simulink model "TST_CrCtl_Governor"  (R2016b)
settings: Solver=FixedStepDiscrete  StartTime=0.0  StopTime=simTime  FixedStep=sampleTime  RelTol=1e-3
values from neighbouring files (symbols this model uses):
  testCase = 1    [initTST_CrCtl_Governor_001.m]    (also in initTST_CrCtl_Governor_002.m = 2; initTST_CrCtl_Governor_003.m = 3; initTST_CrCtl_Governor_004.m = 4; initTST_CrCtl_Governor_005.m = 5)
libraries: simulink x144, UnitTest_Lib x110
(part 7 of 7)

== system TST_CrCtl_Governor/compareSignals/Requirement_002/specifyOutputs ==
  sig_Req_Bus : Inport
  sig_Result_Bus : Inport  Port=2
  AndN : Logic  Inputs=12
  BS_Req : BusSelector  OutputSignals=testSig_CrCtl_rTraV2NBeg,testSig_CrCtl_stOpFunc,testSig_CrCtl_stPtd,testSig_CrCtl_stReq,testSig_CrCtl_stSuspRamp,testSig_CrCtl_stvHysEngBrkReq,testSig_CrCtl_trqLead,testSig_CrCtl_trqLimAct,testSig_CrCtl_trqMin,testSig_CrCtl_trqReq,testSig_CrCtl_trqReqOld,testSig_CrCtl_vMax
  BS_Result : BusSelector  OutputSignals=CrCtl_rTraV2NBeg,CrCtl_stOpFunc,CrCtl_stPtd,CrCtl_stReq,CrCtl_stSuspRamp,CrCtl_stvHysEngBrkReq,CrCtl_trqLead,CrCtl_trqLimAct,CrCtl_trqMin,CrCtl_trqReq,CrCtl_trqReqOld,CrCtl_vMax
  Bitwise_And{1..12} (12 alike) : simulink/Logic and Bit Operations/Bitwise Operator  logicop=AND  UseBitMask=off  BitMask=bin2dec('11011001')  BitMaskRealWorld=Stored Integer
  Relational Operator1 : RelationalOperator  Operator===  OutDataTypeStr=boolean  RndMeth=Simplest
  Relational Operator2 : RelationalOperator  Operator===  OutDataTypeStr=boolean  RndMeth=Simplest
  Scope : Scope  NumInputPorts=12
  Scope{1..12} (12 alike) : Scope  NumInputPorts=2
  cmp_{1,3..4,6..12} (10 alike) : UnitTest_Lib/RoughlyEqual  slope=0.1
  result_tws : ToWorkspace  VariableName=spec_result_002
  tws_1 : ToWorkspace  VariableName=spec_req_002_001
  tws_10 : ToWorkspace  VariableName=spec_req_002_010
  tws_11 : ToWorkspace  VariableName=spec_req_002_011
  tws_12 : ToWorkspace  VariableName=spec_req_002_012
  tws_2 : ToWorkspace  VariableName=spec_req_002_002
  tws_3 : ToWorkspace  VariableName=spec_req_002_003
  tws_4 : ToWorkspace  VariableName=spec_req_002_004
  tws_5 : ToWorkspace  VariableName=spec_req_002_005
  tws_6 : ToWorkspace  VariableName=spec_req_002_006
  tws_7 : ToWorkspace  VariableName=spec_req_002_007
  tws_8 : ToWorkspace  VariableName=spec_req_002_008
  tws_9 : ToWorkspace  VariableName=spec_req_002_009
  result : Outport
  wires:
  sig_Req_Bus/1 -> BS_Req/1
  sig_Result_Bus/1 -> BS_Result/1
  AndN/1 -> result/1, result_tws/1
  BS_Req/1 -> cmp_1/1, Scope1/1  "<testSig_CrCtl_rTraV2NBeg>"
  BS_Result/1 -> cmp_1/2, Scope1/2  "<CrCtl_rTraV2NBeg>"
  cmp_1/1 -> Bitwise_And1/1
  Bitwise_And1/1 -> AndN/1, Scope/1, tws_1/1
  BS_Req/2 -> Relational Operator1/1, Scope2/1  "<testSig_CrCtl_stOpFunc>"
  BS_Result/2 -> Scope2/2, Relational Operator1/2  "<CrCtl_stOpFunc>"
  Relational Operator1/1 -> Bitwise_And2/1
  Bitwise_And2/1 -> AndN/2, Scope/2, tws_2/1
  BS_Req/3 -> cmp_3/1, Scope3/1  "<testSig_CrCtl_stPtd>"
  BS_Result/3 -> cmp_3/2, Scope3/2  "<CrCtl_stPtd>"
  cmp_3/1 -> Bitwise_And3/1
  Bitwise_And3/1 -> AndN/3, Scope/3, tws_3/1
  BS_Req/4 -> cmp_4/1, Scope4/1  "<testSig_CrCtl_stReq>"
  BS_Result/4 -> cmp_4/2, Scope4/2  "<CrCtl_stReq>"
  cmp_4/1 -> Bitwise_And4/1
  Bitwise_And4/1 -> AndN/4, Scope/4, tws_4/1
  BS_Req/5 -> Relational Operator2/1, Scope5/1  "<testSig_CrCtl_stSuspRamp>"
  BS_Result/5 -> Scope5/2, Relational Operator2/2  "<CrCtl_stSuspRamp>"
  Relational Operator2/1 -> Bitwise_And5/1
  Bitwise_And5/1 -> AndN/5, Scope/5, tws_5/1
  BS_Req/6 -> cmp_6/1, Scope6/1  "<testSig_CrCtl_stvHysEngBrkReq>"
  BS_Result/6 -> cmp_6/2, Scope6/2  "<CrCtl_stvHysEngBrkReq>"
  cmp_6/1 -> Bitwise_And6/1
  Bitwise_And6/1 -> AndN/6, Scope/6, tws_6/1
  BS_Req/7 -> cmp_7/1, Scope7/1  "<testSig_CrCtl_trqLead>"
  BS_Result/7 -> cmp_7/2, Scope7/2  "<CrCtl_trqLead>"
  cmp_7/1 -> Bitwise_And7/1
  Bitwise_And7/1 -> AndN/7, Scope/7, tws_7/1
  BS_Req/8 -> cmp_8/1, Scope8/1  "<testSig_CrCtl_trqLimAct>"
  BS_Result/8 -> cmp_8/2, Scope8/2  "<CrCtl_trqLimAct>"
  cmp_8/1 -> Bitwise_And8/1
  Bitwise_And8/1 -> AndN/8, Scope/8, tws_8/1
  BS_Req/9 -> cmp_9/1, Scope9/1  "<testSig_CrCtl_trqMin>"
  BS_Result/9 -> cmp_9/2, Scope9/2  "<CrCtl_trqMin>"
  cmp_9/1 -> Bitwise_And9/1
  Bitwise_And9/1 -> AndN/9, Scope/9, tws_9/1
  BS_Req/10 -> cmp_10/1, Scope10/1  "<testSig_CrCtl_trqReq>"
  BS_Result/10 -> cmp_10/2, Scope10/2  "<CrCtl_trqReq>"
  cmp_10/1 -> Bitwise_And10/1
  Bitwise_And10/1 -> AndN/10, Scope/10, tws_10/1
  BS_Req/11 -> cmp_11/1, Scope11/1  "<testSig_CrCtl_trqReqOld>"
  BS_Result/11 -> cmp_11/2, Scope11/2  "<CrCtl_trqReqOld>"
  cmp_11/1 -> Bitwise_And11/1
  Bitwise_And11/1 -> AndN/11, Scope/11, tws_11/1
  BS_Req/12 -> cmp_12/1, Scope12/1  "<testSig_CrCtl_vMax>"
  BS_Result/12 -> cmp_12/2, Scope12/2  "<CrCtl_vMax>"
  cmp_12/1 -> Bitwise_And12/1
  Bitwise_And12/1 -> AndN/12, Scope/12, tws_12/1

== system TST_CrCtl_Governor/compareSignals/Requirement_003/specifyOutputs ==
  sig_Req_Bus : Inport
  sig_Result_Bus : Inport  Port=2
  AndN : Logic  Inputs=12
  BS_Req : BusSelector  OutputSignals=testSig_CrCtl_rTraV2NBeg,testSig_CrCtl_stOpFunc,testSig_CrCtl_stPtd,testSig_CrCtl_stReq,testSig_CrCtl_stSuspRamp,testSig_CrCtl_stvHysEngBrkReq,testSig_CrCtl_trqLead,testSig_CrCtl_trqLimAct,testSig_CrCtl_trqMin,testSig_CrCtl_trqReq,testSig_CrCtl_trqReqOld,testSig_CrCtl_vMax
  BS_Result : BusSelector  OutputSignals=CrCtl_rTraV2NBeg,CrCtl_stOpFunc,CrCtl_stPtd,CrCtl_stReq,CrCtl_stSuspRamp,CrCtl_stvHysEngBrkReq,CrCtl_trqLead,CrCtl_trqLimAct,CrCtl_trqMin,CrCtl_trqReq,CrCtl_trqReqOld,CrCtl_vMax
  Bitwise_And{1..12} (12 alike) : simulink/Logic and Bit Operations/Bitwise Operator  logicop=AND  UseBitMask=off  BitMask=bin2dec('11011001')  BitMaskRealWorld=Stored Integer
  Relational Operator1 : RelationalOperator  Operator===  OutDataTypeStr=boolean  RndMeth=Simplest
  Relational Operator2 : RelationalOperator  Operator===  OutDataTypeStr=boolean  RndMeth=Simplest
  Scope : Scope  NumInputPorts=12
  Scope{1..12} (12 alike) : Scope  NumInputPorts=2
  cmp_{1,3..4,6..12} (10 alike) : UnitTest_Lib/RoughlyEqual  slope=0.1
  result_tws : ToWorkspace  VariableName=spec_result_003
  tws_1 : ToWorkspace  VariableName=spec_req_003_001
  tws_10 : ToWorkspace  VariableName=spec_req_003_010
  tws_11 : ToWorkspace  VariableName=spec_req_003_011
  tws_12 : ToWorkspace  VariableName=spec_req_003_012
  tws_2 : ToWorkspace  VariableName=spec_req_003_002
  tws_3 : ToWorkspace  VariableName=spec_req_003_003
  tws_4 : ToWorkspace  VariableName=spec_req_003_004
  tws_5 : ToWorkspace  VariableName=spec_req_003_005
  tws_6 : ToWorkspace  VariableName=spec_req_003_006
  tws_7 : ToWorkspace  VariableName=spec_req_003_007
  tws_8 : ToWorkspace  VariableName=spec_req_003_008
  tws_9 : ToWorkspace  VariableName=spec_req_003_009
  result : Outport
  wires:
  sig_Req_Bus/1 -> BS_Req/1
  sig_Result_Bus/1 -> BS_Result/1
  AndN/1 -> result/1, result_tws/1
  BS_Req/1 -> cmp_1/1, Scope1/1  "<testSig_CrCtl_rTraV2NBeg>"
  BS_Result/1 -> cmp_1/2, Scope1/2  "<CrCtl_rTraV2NBeg>"
  cmp_1/1 -> Bitwise_And1/1
  Bitwise_And1/1 -> AndN/1, Scope/1, tws_1/1
  BS_Req/2 -> Relational Operator1/1, Scope2/1  "<testSig_CrCtl_stOpFunc>"
  BS_Result/2 -> Scope2/2, Relational Operator1/2  "<CrCtl_stOpFunc>"
  Relational Operator1/1 -> Bitwise_And2/1
  Bitwise_And2/1 -> AndN/2, Scope/2, tws_2/1
  BS_Req/3 -> cmp_3/1, Scope3/1  "<testSig_CrCtl_stPtd>"
  BS_Result/3 -> cmp_3/2, Scope3/2  "<CrCtl_stPtd>"
  cmp_3/1 -> Bitwise_And3/1
  Bitwise_And3/1 -> AndN/3, Scope/3, tws_3/1
  BS_Req/4 -> cmp_4/1, Scope4/1  "<testSig_CrCtl_stReq>"
  BS_Result/4 -> cmp_4/2, Scope4/2  "<CrCtl_stReq>"
  cmp_4/1 -> Bitwise_And4/1
  Bitwise_And4/1 -> AndN/4, Scope/4, tws_4/1
  BS_Req/5 -> Relational Operator2/1, Scope5/1  "<testSig_CrCtl_stSuspRamp>"
  BS_Result/5 -> Scope5/2, Relational Operator2/2  "<CrCtl_stSuspRamp>"
  Relational Operator2/1 -> Bitwise_And5/1
  Bitwise_And5/1 -> AndN/5, Scope/5, tws_5/1
  BS_Req/6 -> cmp_6/1, Scope6/1  "<testSig_CrCtl_stvHysEngBrkReq>"
  BS_Result/6 -> cmp_6/2, Scope6/2  "<CrCtl_stvHysEngBrkReq>"
  cmp_6/1 -> Bitwise_And6/1
  Bitwise_And6/1 -> AndN/6, Scope/6, tws_6/1
  BS_Req/7 -> cmp_7/1, Scope7/1  "<testSig_CrCtl_trqLead>"
  BS_Result/7 -> cmp_7/2, Scope7/2  "<CrCtl_trqLead>"
  cmp_7/1 -> Bitwise_And7/1
  Bitwise_And7/1 -> AndN/7, Scope/7, tws_7/1
  BS_Req/8 -> cmp_8/1, Scope8/1  "<testSig_CrCtl_trqLimAct>"
  BS_Result/8 -> cmp_8/2, Scope8/2  "<CrCtl_trqLimAct>"
  cmp_8/1 -> Bitwise_And8/1
  Bitwise_And8/1 -> AndN/8, Scope/8, tws_8/1
  BS_Req/9 -> cmp_9/1, Scope9/1  "<testSig_CrCtl_trqMin>"
  BS_Result/9 -> cmp_9/2, Scope9/2  "<CrCtl_trqMin>"
  cmp_9/1 -> Bitwise_And9/1
  Bitwise_And9/1 -> AndN/9, Scope/9, tws_9/1
  BS_Req/10 -> cmp_10/1, Scope10/1  "<testSig_CrCtl_trqReq>"
  BS_Result/10 -> cmp_10/2, Scope10/2  "<CrCtl_trqReq>"
  cmp_10/1 -> Bitwise_And10/1
  Bitwise_And10/1 -> AndN/10, Scope/10, tws_10/1
  BS_Req/11 -> cmp_11/1, Scope11/1  "<testSig_CrCtl_trqReqOld>"
  BS_Result/11 -> cmp_11/2, Scope11/2  "<CrCtl_trqReqOld>"
  cmp_11/1 -> Bitwise_And11/1
  Bitwise_And11/1 -> AndN/11, Scope/11, tws_11/1
  BS_Req/12 -> cmp_12/1, Scope12/1  "<testSig_CrCtl_vMax>"
  BS_Result/12 -> cmp_12/2, Scope12/2  "<CrCtl_vMax>"
  cmp_12/1 -> Bitwise_And12/1
  Bitwise_And12/1 -> AndN/12, Scope/12, tws_12/1

== system TST_CrCtl_Governor/compareSignals/Requirement_004/specifyOutputs ==
  sig_Req_Bus : Inport
  sig_Result_Bus : Inport  Port=2
  AndN : Logic  Inputs=12
  BS_Req : BusSelector  OutputSignals=testSig_CrCtl_rTraV2NBeg,testSig_CrCtl_stOpFunc,testSig_CrCtl_stPtd,testSig_CrCtl_stReq,testSig_CrCtl_stSuspRamp,testSig_CrCtl_stvHysEngBrkReq,testSig_CrCtl_trqLead,testSig_CrCtl_trqLimAct,testSig_CrCtl_trqMin,testSig_CrCtl_trqReq,testSig_CrCtl_trqReqOld,testSig_CrCtl_vMax
  BS_Result : BusSelector  OutputSignals=CrCtl_rTraV2NBeg,CrCtl_stOpFunc,CrCtl_stPtd,CrCtl_stReq,CrCtl_stSuspRamp,CrCtl_stvHysEngBrkReq,CrCtl_trqLead,CrCtl_trqLimAct,CrCtl_trqMin,CrCtl_trqReq,CrCtl_trqReqOld,CrCtl_vMax
  Bitwise_And{1..12} (12 alike) : simulink/Logic and Bit Operations/Bitwise Operator  logicop=AND  UseBitMask=off  BitMask=bin2dec('11011001')  BitMaskRealWorld=Stored Integer
  Relational Operator1 : RelationalOperator  Operator===  OutDataTypeStr=boolean  RndMeth=Simplest
  Relational Operator2 : RelationalOperator  Operator===  OutDataTypeStr=boolean  RndMeth=Simplest
  Scope : Scope  NumInputPorts=12
  Scope{1..12} (12 alike) : Scope  NumInputPorts=2
  cmp_{1,3..4,6..12} (10 alike) : UnitTest_Lib/RoughlyEqual  slope=0.1
  result_tws : ToWorkspace  VariableName=spec_result_004
  tws_1 : ToWorkspace  VariableName=spec_req_004_001
  tws_10 : ToWorkspace  VariableName=spec_req_004_010
  tws_11 : ToWorkspace  VariableName=spec_req_004_011
  tws_12 : ToWorkspace  VariableName=spec_req_004_012
  tws_2 : ToWorkspace  VariableName=spec_req_004_002
  tws_3 : ToWorkspace  VariableName=spec_req_004_003
  tws_4 : ToWorkspace  VariableName=spec_req_004_004
  tws_5 : ToWorkspace  VariableName=spec_req_004_005
  tws_6 : ToWorkspace  VariableName=spec_req_004_006
  tws_7 : ToWorkspace  VariableName=spec_req_004_007
  tws_8 : ToWorkspace  VariableName=spec_req_004_008
  tws_9 : ToWorkspace  VariableName=spec_req_004_009
  result : Outport
  wires:
  sig_Req_Bus/1 -> BS_Req/1
  sig_Result_Bus/1 -> BS_Result/1
  AndN/1 -> result/1, result_tws/1
  BS_Req/1 -> cmp_1/1, Scope1/1  "<testSig_CrCtl_rTraV2NBeg>"
  BS_Result/1 -> cmp_1/2, Scope1/2  "<CrCtl_rTraV2NBeg>"
  cmp_1/1 -> Bitwise_And1/1
  Bitwise_And1/1 -> AndN/1, Scope/1, tws_1/1
  BS_Req/2 -> Relational Operator1/1, Scope2/1  "<testSig_CrCtl_stOpFunc>"
  BS_Result/2 -> Relational Operator1/2, Scope2/2  "<CrCtl_stOpFunc>"
  Relational Operator1/1 -> Bitwise_And2/1
  Bitwise_And2/1 -> AndN/2, Scope/2, tws_2/1
  BS_Req/3 -> cmp_3/1, Scope3/1  "<testSig_CrCtl_stPtd>"
  BS_Result/3 -> cmp_3/2, Scope3/2  "<CrCtl_stPtd>"
  cmp_3/1 -> Bitwise_And3/1
  Bitwise_And3/1 -> AndN/3, Scope/3, tws_3/1
  BS_Req/4 -> cmp_4/1, Scope4/1  "<testSig_CrCtl_stReq>"
  BS_Result/4 -> cmp_4/2, Scope4/2  "<CrCtl_stReq>"
  cmp_4/1 -> Bitwise_And4/1
  Bitwise_And4/1 -> AndN/4, Scope/4, tws_4/1
  BS_Req/5 -> Relational Operator2/1, Scope5/1  "<testSig_CrCtl_stSuspRamp>"
  BS_Result/5 -> Scope5/2, Relational Operator2/2  "<CrCtl_stSuspRamp>"
  Relational Operator2/1 -> Bitwise_And5/1
  Bitwise_And5/1 -> AndN/5, Scope/5, tws_5/1
  BS_Req/6 -> cmp_6/1, Scope6/1  "<testSig_CrCtl_stvHysEngBrkReq>"
  BS_Result/6 -> cmp_6/2, Scope6/2  "<CrCtl_stvHysEngBrkReq>"
  cmp_6/1 -> Bitwise_And6/1
  Bitwise_And6/1 -> AndN/6, Scope/6, tws_6/1
  BS_Req/7 -> cmp_7/1, Scope7/1  "<testSig_CrCtl_trqLead>"
  BS_Result/7 -> cmp_7/2, Scope7/2  "<CrCtl_trqLead>"
  cmp_7/1 -> Bitwise_And7/1
  Bitwise_And7/1 -> AndN/7, Scope/7, tws_7/1
  BS_Req/8 -> cmp_8/1, Scope8/1  "<testSig_CrCtl_trqLimAct>"
  BS_Result/8 -> cmp_8/2, Scope8/2  "<CrCtl_trqLimAct>"
  cmp_8/1 -> Bitwise_And8/1
  Bitwise_And8/1 -> AndN/8, Scope/8, tws_8/1
  BS_Req/9 -> cmp_9/1, Scope9/1  "<testSig_CrCtl_trqMin>"
  BS_Result/9 -> cmp_9/2, Scope9/2  "<CrCtl_trqMin>"
  cmp_9/1 -> Bitwise_And9/1
  Bitwise_And9/1 -> AndN/9, Scope/9, tws_9/1
  BS_Req/10 -> cmp_10/1, Scope10/1  "<testSig_CrCtl_trqReq>"
  BS_Result/10 -> cmp_10/2, Scope10/2  "<CrCtl_trqReq>"
  cmp_10/1 -> Bitwise_And10/1
  Bitwise_And10/1 -> AndN/10, Scope/10, tws_10/1
  BS_Req/11 -> cmp_11/1, Scope11/1  "<testSig_CrCtl_trqReqOld>"
  BS_Result/11 -> cmp_11/2, Scope11/2  "<CrCtl_trqReqOld>"
  cmp_11/1 -> Bitwise_And11/1
  Bitwise_And11/1 -> AndN/11, Scope/11, tws_11/1
  BS_Req/12 -> cmp_12/1, Scope12/1  "<testSig_CrCtl_vMax>"
  BS_Result/12 -> cmp_12/2, Scope12/2  "<CrCtl_vMax>"
  cmp_12/1 -> Bitwise_And12/1
  Bitwise_And12/1 -> AndN/12, Scope/12, tws_12/1

== system TST_CrCtl_Governor/compareSignals/Requirement_005/specifyOutputs ==
  sig_Req_Bus : Inport
  sig_Result_Bus : Inport  Port=2
  AndN : Logic  Inputs=12
  BS_Req : BusSelector  OutputSignals=testSig_CrCtl_rTraV2NBeg,testSig_CrCtl_stOpFunc,testSig_CrCtl_stPtd,testSig_CrCtl_stReq,testSig_CrCtl_stSuspRamp,testSig_CrCtl_stvHysEngBrkReq,testSig_CrCtl_trqLead,testSig_CrCtl_trqLimAct,testSig_CrCtl_trqMin,testSig_CrCtl_trqReq,testSig_CrCtl_trqReqOld,testSig_CrCtl_vMax
  BS_Result : BusSelector  OutputSignals=CrCtl_rTraV2NBeg,CrCtl_stOpFunc,CrCtl_stPtd,CrCtl_stReq,CrCtl_stSuspRamp,CrCtl_stvHysEngBrkReq,CrCtl_trqLead,CrCtl_trqLimAct,CrCtl_trqMin,CrCtl_trqReq,CrCtl_trqReqOld,CrCtl_vMax
  Bitwise_And{1..12} (12 alike) : simulink/Logic and Bit Operations/Bitwise Operator  logicop=AND  UseBitMask=off  BitMask=bin2dec('11011001')  BitMaskRealWorld=Stored Integer
  Relational Operator1 : RelationalOperator  Operator===  OutDataTypeStr=boolean  RndMeth=Simplest
  Relational Operator2 : RelationalOperator  Operator===  OutDataTypeStr=boolean  RndMeth=Simplest
  Scope : Scope  NumInputPorts=12
  Scope{1..12} (12 alike) : Scope  NumInputPorts=2
  cmp_{1,3..4,6..9,12} (8 alike) : UnitTest_Lib/RoughlyEqual  slope=0.1
  cmp_10 : UnitTest_Lib/RoughlyEqual  slope=0.5
  cmp_11 : UnitTest_Lib/RoughlyEqual  slope=0.5
  result_tws : ToWorkspace  VariableName=spec_result_005
  tws_1 : ToWorkspace  VariableName=spec_req_005_001
  tws_10 : ToWorkspace  VariableName=spec_req_005_010
  tws_11 : ToWorkspace  VariableName=spec_req_005_011
  tws_12 : ToWorkspace  VariableName=spec_req_005_012
  tws_2 : ToWorkspace  VariableName=spec_req_005_002
  tws_3 : ToWorkspace  VariableName=spec_req_005_003
  tws_4 : ToWorkspace  VariableName=spec_req_005_004
  tws_5 : ToWorkspace  VariableName=spec_req_005_005
  tws_6 : ToWorkspace  VariableName=spec_req_005_006
  tws_7 : ToWorkspace  VariableName=spec_req_005_007
  tws_8 : ToWorkspace  VariableName=spec_req_005_008
  tws_9 : ToWorkspace  VariableName=spec_req_005_009
  result : Outport
  wires:
  sig_Req_Bus/1 -> BS_Req/1
  sig_Result_Bus/1 -> BS_Result/1
  AndN/1 -> result/1, result_tws/1
  BS_Req/1 -> cmp_1/1, Scope1/1  "<testSig_CrCtl_rTraV2NBeg>"
  BS_Result/1 -> cmp_1/2, Scope1/2  "<CrCtl_rTraV2NBeg>"
  cmp_1/1 -> Bitwise_And1/1
  Bitwise_And1/1 -> AndN/1, Scope/1, tws_1/1
  BS_Req/2 -> Relational Operator1/1, Scope2/1  "<testSig_CrCtl_stOpFunc>"
  BS_Result/2 -> Relational Operator1/2, Scope2/2  "<CrCtl_stOpFunc>"
  Relational Operator1/1 -> Bitwise_And2/1
  Bitwise_And2/1 -> AndN/2, Scope/2, tws_2/1
  BS_Req/3 -> cmp_3/1, Scope3/1  "<testSig_CrCtl_stPtd>"
  BS_Result/3 -> cmp_3/2, Scope3/2  "<CrCtl_stPtd>"
  cmp_3/1 -> Bitwise_And3/1
  Bitwise_And3/1 -> AndN/3, Scope/3, tws_3/1
  BS_Req/4 -> cmp_4/1, Scope4/1  "<testSig_CrCtl_stReq>"
  BS_Result/4 -> cmp_4/2, Scope4/2  "<CrCtl_stReq>"
  cmp_4/1 -> Bitwise_And4/1
  Bitwise_And4/1 -> AndN/4, Scope/4, tws_4/1
  BS_Req/5 -> Relational Operator2/1, Scope5/1  "<testSig_CrCtl_stSuspRamp>"
  BS_Result/5 -> Scope5/2, Relational Operator2/2  "<CrCtl_stSuspRamp>"
  Relational Operator2/1 -> Bitwise_And5/1
  Bitwise_And5/1 -> AndN/5, Scope/5, tws_5/1
  BS_Req/6 -> cmp_6/1, Scope6/1  "<testSig_CrCtl_stvHysEngBrkReq>"
  BS_Result/6 -> cmp_6/2, Scope6/2  "<CrCtl_stvHysEngBrkReq>"
  cmp_6/1 -> Bitwise_And6/1
  Bitwise_And6/1 -> AndN/6, Scope/6, tws_6/1
  BS_Req/7 -> cmp_7/1, Scope7/1  "<testSig_CrCtl_trqLead>"
  BS_Result/7 -> cmp_7/2, Scope7/2  "<CrCtl_trqLead>"
  cmp_7/1 -> Bitwise_And7/1
  Bitwise_And7/1 -> AndN/7, Scope/7, tws_7/1
  BS_Req/8 -> cmp_8/1, Scope8/1  "<testSig_CrCtl_trqLimAct>"
  BS_Result/8 -> cmp_8/2, Scope8/2  "<CrCtl_trqLimAct>"
  cmp_8/1 -> Bitwise_And8/1
  Bitwise_And8/1 -> AndN/8, Scope/8, tws_8/1
  BS_Req/9 -> cmp_9/1, Scope9/1  "<testSig_CrCtl_trqMin>"
  BS_Result/9 -> cmp_9/2, Scope9/2  "<CrCtl_trqMin>"
  cmp_9/1 -> Bitwise_And9/1
  Bitwise_And9/1 -> AndN/9, Scope/9, tws_9/1
  BS_Req/10 -> cmp_10/1, Scope10/1  "<testSig_CrCtl_trqReq>"
  BS_Result/10 -> cmp_10/2, Scope10/2  "<CrCtl_trqReq>"
  cmp_10/1 -> Bitwise_And10/1
  Bitwise_And10/1 -> AndN/10, Scope/10, tws_10/1
  BS_Req/11 -> cmp_11/1, Scope11/1  "<testSig_CrCtl_trqReqOld>"
  BS_Result/11 -> cmp_11/2, Scope11/2  "<CrCtl_trqReqOld>"
  cmp_11/1 -> Bitwise_And11/1
  Bitwise_And11/1 -> AndN/11, Scope/11, tws_11/1
  BS_Req/12 -> cmp_12/1, Scope12/1  "<testSig_CrCtl_vMax>"
  BS_Result/12 -> cmp_12/2, Scope12/2  "<CrCtl_vMax>"
  cmp_12/1 -> Bitwise_And12/1
  Bitwise_And12/1 -> AndN/12, Scope/12, tws_12/1

== system TST_CrCtl_Governor/compareSignals/Requirement_006/specifyOutputs ==
  sig_Req_Bus : Inport
  sig_Result_Bus : Inport  Port=2
  AndN : Logic  Inputs=12
  BS_Req : BusSelector  OutputSignals=testSig_CrCtl_rTraV2NBeg,testSig_CrCtl_stOpFunc,testSig_CrCtl_stPtd,testSig_CrCtl_stReq,testSig_CrCtl_stSuspRamp,testSig_CrCtl_stvHysEngBrkReq,testSig_CrCtl_trqLead,testSig_CrCtl_trqLimAct,testSig_CrCtl_trqMin,testSig_CrCtl_trqReq,testSig_CrCtl_trqReqOld,testSig_CrCtl_vMax
  BS_Result : BusSelector  OutputSignals=CrCtl_rTraV2NBeg,CrCtl_stOpFunc,CrCtl_stPtd,CrCtl_stReq,CrCtl_stSuspRamp,CrCtl_stvHysEngBrkReq,CrCtl_trqLead,CrCtl_trqLimAct,CrCtl_trqMin,CrCtl_trqReq,CrCtl_trqReqOld,CrCtl_vMax
  Bitwise_And{1..12} (12 alike) : simulink/Logic and Bit Operations/Bitwise Operator  logicop=AND  UseBitMask=off  BitMask=bin2dec('11011001')  BitMaskRealWorld=Stored Integer
  Relational Operator1 : RelationalOperator  Operator===  OutDataTypeStr=boolean  RndMeth=Simplest
  Relational Operator2 : RelationalOperator  Operator===  OutDataTypeStr=boolean  RndMeth=Simplest
  Scope : Scope  NumInputPorts=12
  Scope{1..12} (12 alike) : Scope  NumInputPorts=2
  cmp_{1,3..4,6..12} (10 alike) : UnitTest_Lib/RoughlyEqual  slope=0.1
  result_tws : ToWorkspace  VariableName=spec_result_006
  tws_1 : ToWorkspace  VariableName=spec_req_006_001
  tws_10 : ToWorkspace  VariableName=spec_req_006_010
  tws_11 : ToWorkspace  VariableName=spec_req_006_011
  tws_12 : ToWorkspace  VariableName=spec_req_006_012
  tws_2 : ToWorkspace  VariableName=spec_req_006_002
  tws_3 : ToWorkspace  VariableName=spec_req_006_003
  tws_4 : ToWorkspace  VariableName=spec_req_006_004
  tws_5 : ToWorkspace  VariableName=spec_req_006_005
  tws_6 : ToWorkspace  VariableName=spec_req_006_006
  tws_7 : ToWorkspace  VariableName=spec_req_006_007
  tws_8 : ToWorkspace  VariableName=spec_req_006_008
  tws_9 : ToWorkspace  VariableName=spec_req_006_009
  result : Outport
  wires:
  sig_Req_Bus/1 -> BS_Req/1
  sig_Result_Bus/1 -> BS_Result/1
  AndN/1 -> result/1, result_tws/1
  BS_Req/1 -> cmp_1/1, Scope1/1  "<testSig_CrCtl_rTraV2NBeg>"
  BS_Result/1 -> cmp_1/2, Scope1/2  "<CrCtl_rTraV2NBeg>"
  cmp_1/1 -> Bitwise_And1/1
  Bitwise_And1/1 -> AndN/1, Scope/1, tws_1/1
  BS_Req/2 -> Relational Operator1/1, Scope2/1  "<testSig_CrCtl_stOpFunc>"
  BS_Result/2 -> Scope2/2, Relational Operator1/2  "<CrCtl_stOpFunc>"
  Relational Operator1/1 -> Bitwise_And2/1
  Bitwise_And2/1 -> AndN/2, Scope/2, tws_2/1
  BS_Req/3 -> cmp_3/1, Scope3/1  "<testSig_CrCtl_stPtd>"
  BS_Result/3 -> cmp_3/2, Scope3/2  "<CrCtl_stPtd>"
  cmp_3/1 -> Bitwise_And3/1
  Bitwise_And3/1 -> AndN/3, Scope/3, tws_3/1
  BS_Req/4 -> cmp_4/1, Scope4/1  "<testSig_CrCtl_stReq>"
  BS_Result/4 -> cmp_4/2, Scope4/2  "<CrCtl_stReq>"
  cmp_4/1 -> Bitwise_And4/1
  Bitwise_And4/1 -> AndN/4, Scope/4, tws_4/1
  BS_Req/5 -> Relational Operator2/1, Scope5/1  "<testSig_CrCtl_stSuspRamp>"
  BS_Result/5 -> Relational Operator2/2, Scope5/2  "<CrCtl_stSuspRamp>"
  Relational Operator2/1 -> Bitwise_And5/1
  Bitwise_And5/1 -> AndN/5, Scope/5, tws_5/1
  BS_Req/6 -> cmp_6/1, Scope6/1  "<testSig_CrCtl_stvHysEngBrkReq>"
  BS_Result/6 -> cmp_6/2, Scope6/2  "<CrCtl_stvHysEngBrkReq>"
  cmp_6/1 -> Bitwise_And6/1
  Bitwise_And6/1 -> AndN/6, Scope/6, tws_6/1
  BS_Req/7 -> cmp_7/1, Scope7/1  "<testSig_CrCtl_trqLead>"
  BS_Result/7 -> cmp_7/2, Scope7/2  "<CrCtl_trqLead>"
  cmp_7/1 -> Bitwise_And7/1
  Bitwise_And7/1 -> AndN/7, Scope/7, tws_7/1
  BS_Req/8 -> cmp_8/1, Scope8/1  "<testSig_CrCtl_trqLimAct>"
  BS_Result/8 -> cmp_8/2, Scope8/2  "<CrCtl_trqLimAct>"
  cmp_8/1 -> Bitwise_And8/1
  Bitwise_And8/1 -> AndN/8, Scope/8, tws_8/1
  BS_Req/9 -> cmp_9/1, Scope9/1  "<testSig_CrCtl_trqMin>"
  BS_Result/9 -> cmp_9/2, Scope9/2  "<CrCtl_trqMin>"
  cmp_9/1 -> Bitwise_And9/1
  Bitwise_And9/1 -> AndN/9, Scope/9, tws_9/1
  BS_Req/10 -> cmp_10/1, Scope10/1  "<testSig_CrCtl_trqReq>"
  BS_Result/10 -> cmp_10/2, Scope10/2  "<CrCtl_trqReq>"
  cmp_10/1 -> Bitwise_And10/1
  Bitwise_And10/1 -> AndN/10, Scope/10, tws_10/1
  BS_Req/11 -> cmp_11/1, Scope11/1  "<testSig_CrCtl_trqReqOld>"
  BS_Result/11 -> cmp_11/2, Scope11/2  "<CrCtl_trqReqOld>"
  cmp_11/1 -> Bitwise_And11/1
  Bitwise_And11/1 -> AndN/11, Scope/11, tws_11/1
  BS_Req/12 -> cmp_12/1, Scope12/1  "<testSig_CrCtl_vMax>"
  BS_Result/12 -> cmp_12/2, Scope12/2  "<CrCtl_vMax>"
  cmp_12/1 -> Bitwise_And12/1
  Bitwise_And12/1 -> AndN/12, Scope/12, tws_12/1

== system TST_CrCtl_Governor/compareSignals/Requirement_007/specifyOutputs ==
  sig_Req_Bus : Inport
  sig_Result_Bus : Inport  Port=2
  AndN : Logic  Inputs=12
  BS_Req : BusSelector  OutputSignals=testSig_CrCtl_rTraV2NBeg,testSig_CrCtl_stOpFunc,testSig_CrCtl_stPtd,testSig_CrCtl_stReq,testSig_CrCtl_stSuspRamp,testSig_CrCtl_stvHysEngBrkReq,testSig_CrCtl_trqLead,testSig_CrCtl_trqLimAct,testSig_CrCtl_trqMin,testSig_CrCtl_trqReq,testSig_CrCtl_trqReqOld,testSig_CrCtl_vMax
  BS_Result : BusSelector  OutputSignals=CrCtl_rTraV2NBeg,CrCtl_stOpFunc,CrCtl_stPtd,CrCtl_stReq,CrCtl_stSuspRamp,CrCtl_stvHysEngBrkReq,CrCtl_trqLead,CrCtl_trqLimAct,CrCtl_trqMin,CrCtl_trqReq,CrCtl_trqReqOld,CrCtl_vMax
  Bitwise_And{1..12} (12 alike) : simulink/Logic and Bit Operations/Bitwise Operator  logicop=AND  UseBitMask=off  BitMask=bin2dec('11011001')  BitMaskRealWorld=Stored Integer
  Relational Operator1 : RelationalOperator  Operator===  OutDataTypeStr=boolean  RndMeth=Simplest
  Relational Operator2 : RelationalOperator  Operator===  OutDataTypeStr=boolean  RndMeth=Simplest
  Scope : Scope  NumInputPorts=12
  Scope{1..12} (12 alike) : Scope  NumInputPorts=2
  cmp_{1,3..4,6..12} (10 alike) : UnitTest_Lib/RoughlyEqual  slope=0.1
  result_tws : ToWorkspace  VariableName=spec_result_007
  tws_1 : ToWorkspace  VariableName=spec_req_007_001
  tws_10 : ToWorkspace  VariableName=spec_req_007_010
  tws_11 : ToWorkspace  VariableName=spec_req_007_011
  tws_12 : ToWorkspace  VariableName=spec_req_007_012
  tws_2 : ToWorkspace  VariableName=spec_req_007_002
  tws_3 : ToWorkspace  VariableName=spec_req_007_003
  tws_4 : ToWorkspace  VariableName=spec_req_007_004
  tws_5 : ToWorkspace  VariableName=spec_req_007_005
  tws_6 : ToWorkspace  VariableName=spec_req_007_006
  tws_7 : ToWorkspace  VariableName=spec_req_007_007
  tws_8 : ToWorkspace  VariableName=spec_req_007_008
  tws_9 : ToWorkspace  VariableName=spec_req_007_009
  result : Outport
  wires:
  sig_Req_Bus/1 -> BS_Req/1
  sig_Result_Bus/1 -> BS_Result/1
  AndN/1 -> result/1, result_tws/1
  BS_Req/1 -> cmp_1/1, Scope1/1  "<testSig_CrCtl_rTraV2NBeg>"
  BS_Result/1 -> cmp_1/2, Scope1/2  "<CrCtl_rTraV2NBeg>"
  cmp_1/1 -> Bitwise_And1/1
  Bitwise_And1/1 -> AndN/1, Scope/1, tws_1/1
  BS_Req/2 -> Relational Operator1/1, Scope2/1  "<testSig_CrCtl_stOpFunc>"
  BS_Result/2 -> Scope2/2, Relational Operator1/2  "<CrCtl_stOpFunc>"
  Relational Operator1/1 -> Bitwise_And2/1
  Bitwise_And2/1 -> AndN/2, Scope/2, tws_2/1
  BS_Req/3 -> cmp_3/1, Scope3/1  "<testSig_CrCtl_stPtd>"
  BS_Result/3 -> cmp_3/2, Scope3/2  "<CrCtl_stPtd>"
  cmp_3/1 -> Bitwise_And3/1
  Bitwise_And3/1 -> AndN/3, Scope/3, tws_3/1
  BS_Req/4 -> cmp_4/1, Scope4/1  "<testSig_CrCtl_stReq>"
  BS_Result/4 -> cmp_4/2, Scope4/2  "<CrCtl_stReq>"
  cmp_4/1 -> Bitwise_And4/1
  Bitwise_And4/1 -> AndN/4, Scope/4, tws_4/1
  BS_Req/5 -> Relational Operator2/1, Scope5/1  "<testSig_CrCtl_stSuspRamp>"
  BS_Result/5 -> Scope5/2, Relational Operator2/2  "<CrCtl_stSuspRamp>"
  Relational Operator2/1 -> Bitwise_And5/1
  Bitwise_And5/1 -> AndN/5, Scope/5, tws_5/1
  BS_Req/6 -> cmp_6/1, Scope6/1  "<testSig_CrCtl_stvHysEngBrkReq>"
  BS_Result/6 -> cmp_6/2, Scope6/2  "<CrCtl_stvHysEngBrkReq>"
  cmp_6/1 -> Bitwise_And6/1
  Bitwise_And6/1 -> AndN/6, Scope/6, tws_6/1
  BS_Req/7 -> cmp_7/1, Scope7/1  "<testSig_CrCtl_trqLead>"
  BS_Result/7 -> cmp_7/2, Scope7/2  "<CrCtl_trqLead>"
  cmp_7/1 -> Bitwise_And7/1
  Bitwise_And7/1 -> AndN/7, Scope/7, tws_7/1
  BS_Req/8 -> cmp_8/1, Scope8/1  "<testSig_CrCtl_trqLimAct>"
  BS_Result/8 -> cmp_8/2, Scope8/2  "<CrCtl_trqLimAct>"
  cmp_8/1 -> Bitwise_And8/1
  Bitwise_And8/1 -> AndN/8, Scope/8, tws_8/1
  BS_Req/9 -> cmp_9/1, Scope9/1  "<testSig_CrCtl_trqMin>"
  BS_Result/9 -> cmp_9/2, Scope9/2  "<CrCtl_trqMin>"
  cmp_9/1 -> Bitwise_And9/1
  Bitwise_And9/1 -> AndN/9, Scope/9, tws_9/1
  BS_Req/10 -> cmp_10/1, Scope10/1  "<testSig_CrCtl_trqReq>"
  BS_Result/10 -> cmp_10/2, Scope10/2  "<CrCtl_trqReq>"
  cmp_10/1 -> Bitwise_And10/1
  Bitwise_And10/1 -> AndN/10, Scope/10, tws_10/1
  BS_Req/11 -> cmp_11/1, Scope11/1  "<testSig_CrCtl_trqReqOld>"
  BS_Result/11 -> cmp_11/2, Scope11/2  "<CrCtl_trqReqOld>"
  cmp_11/1 -> Bitwise_And11/1
  Bitwise_And11/1 -> AndN/11, Scope/11, tws_11/1
  BS_Req/12 -> cmp_12/1, Scope12/1  "<testSig_CrCtl_vMax>"
  BS_Result/12 -> cmp_12/2, Scope12/2  "<CrCtl_vMax>"
  cmp_12/1 -> Bitwise_And12/1
  Bitwise_And12/1 -> AndN/12, Scope/12, tws_12/1

== system TST_CrCtl_Governor/compareSignals/Requirement_008/specifyOutputs ==
  sig_Req_Bus : Inport
  sig_Result_Bus : Inport  Port=2
  AndN : Logic  Inputs=12
  BS_Req : BusSelector  OutputSignals=testSig_CrCtl_rTraV2NBeg,testSig_CrCtl_stOpFunc,testSig_CrCtl_stPtd,testSig_CrCtl_stReq,testSig_CrCtl_stSuspRamp,testSig_CrCtl_stvHysEngBrkReq,testSig_CrCtl_trqLead,testSig_CrCtl_trqLimAct,testSig_CrCtl_trqMin,testSig_CrCtl_trqReq,testSig_CrCtl_trqReqOld,testSig_CrCtl_vMax
  BS_Result : BusSelector  OutputSignals=CrCtl_rTraV2NBeg,CrCtl_stOpFunc,CrCtl_stPtd,CrCtl_stReq,CrCtl_stSuspRamp,CrCtl_stvHysEngBrkReq,CrCtl_trqLead,CrCtl_trqLimAct,CrCtl_trqMin,CrCtl_trqReq,CrCtl_trqReqOld,CrCtl_vMax
  Bitwise_And{1..12} (12 alike) : simulink/Logic and Bit Operations/Bitwise Operator  logicop=AND  UseBitMask=off  BitMask=bin2dec('11011001')  BitMaskRealWorld=Stored Integer
  Relational Operator1 : RelationalOperator  Operator===  OutDataTypeStr=boolean  RndMeth=Simplest
  Relational Operator2 : RelationalOperator  Operator===  OutDataTypeStr=boolean  RndMeth=Simplest
  Scope : Scope  NumInputPorts=12
  Scope{1..12} (12 alike) : Scope  NumInputPorts=2
  cmp_{1,3..4,6..12} (10 alike) : UnitTest_Lib/RoughlyEqual  slope=0.1
  result_tws : ToWorkspace  VariableName=spec_result_008
  tws_1 : ToWorkspace  VariableName=spec_req_008_001
  tws_10 : ToWorkspace  VariableName=spec_req_008_010
  tws_11 : ToWorkspace  VariableName=spec_req_008_011
  tws_12 : ToWorkspace  VariableName=spec_req_008_012
  tws_2 : ToWorkspace  VariableName=spec_req_008_002
  tws_3 : ToWorkspace  VariableName=spec_req_008_003
  tws_4 : ToWorkspace  VariableName=spec_req_008_004
  tws_5 : ToWorkspace  VariableName=spec_req_008_005
  tws_6 : ToWorkspace  VariableName=spec_req_008_006
  tws_7 : ToWorkspace  VariableName=spec_req_008_007
  tws_8 : ToWorkspace  VariableName=spec_req_008_008
  tws_9 : ToWorkspace  VariableName=spec_req_008_009
  result : Outport
  wires:
  sig_Req_Bus/1 -> BS_Req/1
  sig_Result_Bus/1 -> BS_Result/1
  AndN/1 -> result/1, result_tws/1
  BS_Req/1 -> cmp_1/1, Scope1/1  "<testSig_CrCtl_rTraV2NBeg>"
  BS_Result/1 -> cmp_1/2, Scope1/2  "<CrCtl_rTraV2NBeg>"
  cmp_1/1 -> Bitwise_And1/1
  Bitwise_And1/1 -> AndN/1, Scope/1, tws_1/1
  BS_Req/2 -> Relational Operator1/1, Scope2/1  "<testSig_CrCtl_stOpFunc>"
  BS_Result/2 -> Relational Operator1/2, Scope2/2  "<CrCtl_stOpFunc>"
  Relational Operator1/1 -> Bitwise_And2/1
  Bitwise_And2/1 -> AndN/2, Scope/2, tws_2/1
  BS_Req/3 -> cmp_3/1, Scope3/1  "<testSig_CrCtl_stPtd>"
  BS_Result/3 -> cmp_3/2, Scope3/2  "<CrCtl_stPtd>"
  cmp_3/1 -> Bitwise_And3/1
  Bitwise_And3/1 -> AndN/3, Scope/3, tws_3/1
  BS_Req/4 -> cmp_4/1, Scope4/1  "<testSig_CrCtl_stReq>"
  BS_Result/4 -> cmp_4/2, Scope4/2  "<CrCtl_stReq>"
  cmp_4/1 -> Bitwise_And4/1
  Bitwise_And4/1 -> AndN/4, Scope/4, tws_4/1
  BS_Req/5 -> Relational Operator2/1, Scope5/1  "<testSig_CrCtl_stSuspRamp>"
  BS_Result/5 -> Relational Operator2/2, Scope5/2  "<CrCtl_stSuspRamp>"
  Relational Operator2/1 -> Bitwise_And5/1
  Bitwise_And5/1 -> AndN/5, Scope/5, tws_5/1
  BS_Req/6 -> cmp_6/1, Scope6/1  "<testSig_CrCtl_stvHysEngBrkReq>"
  BS_Result/6 -> cmp_6/2, Scope6/2  "<CrCtl_stvHysEngBrkReq>"
  cmp_6/1 -> Bitwise_And6/1
  Bitwise_And6/1 -> AndN/6, Scope/6, tws_6/1
  BS_Req/7 -> cmp_7/1, Scope7/1  "<testSig_CrCtl_trqLead>"
  BS_Result/7 -> cmp_7/2, Scope7/2  "<CrCtl_trqLead>"
  cmp_7/1 -> Bitwise_And7/1
  Bitwise_And7/1 -> AndN/7, Scope/7, tws_7/1
  BS_Req/8 -> cmp_8/1, Scope8/1  "<testSig_CrCtl_trqLimAct>"
  BS_Result/8 -> cmp_8/2, Scope8/2  "<CrCtl_trqLimAct>"
  cmp_8/1 -> Bitwise_And8/1
  Bitwise_And8/1 -> AndN/8, Scope/8, tws_8/1
  BS_Req/9 -> cmp_9/1, Scope9/1  "<testSig_CrCtl_trqMin>"
  BS_Result/9 -> cmp_9/2, Scope9/2  "<CrCtl_trqMin>"
  cmp_9/1 -> Bitwise_And9/1
  Bitwise_And9/1 -> AndN/9, Scope/9, tws_9/1
  BS_Req/10 -> cmp_10/1, Scope10/1  "<testSig_CrCtl_trqReq>"
  BS_Result/10 -> cmp_10/2, Scope10/2  "<CrCtl_trqReq>"
  cmp_10/1 -> Bitwise_And10/1
  Bitwise_And10/1 -> AndN/10, Scope/10, tws_10/1
  BS_Req/11 -> cmp_11/1, Scope11/1  "<testSig_CrCtl_trqReqOld>"
  BS_Result/11 -> cmp_11/2, Scope11/2  "<CrCtl_trqReqOld>"
  cmp_11/1 -> Bitwise_And11/1
  Bitwise_And11/1 -> AndN/11, Scope/11, tws_11/1
  BS_Req/12 -> cmp_12/1, Scope12/1  "<testSig_CrCtl_vMax>"
  BS_Result/12 -> cmp_12/2, Scope12/2  "<CrCtl_vMax>"
  cmp_12/1 -> Bitwise_And12/1
  Bitwise_And12/1 -> AndN/12, Scope/12, tws_12/1

== system TST_CrCtl_Governor/compareSignals/Requirement_009/specifyOutputs ==
  sig_Req_Bus : Inport
  sig_Result_Bus : Inport  Port=2
  AndN : Logic  Inputs=12
  BS_Req : BusSelector  OutputSignals=testSig_CrCtl_rTraV2NBeg,testSig_CrCtl_stOpFunc,testSig_CrCtl_stPtd,testSig_CrCtl_stReq,testSig_CrCtl_stSuspRamp,testSig_CrCtl_stvHysEngBrkReq,testSig_CrCtl_trqLead,testSig_CrCtl_trqLimAct,testSig_CrCtl_trqMin,testSig_CrCtl_trqReq,testSig_CrCtl_trqReqOld,testSig_CrCtl_vMax
  BS_Result : BusSelector  OutputSignals=CrCtl_rTraV2NBeg,CrCtl_stOpFunc,CrCtl_stPtd,CrCtl_stReq,CrCtl_stSuspRamp,CrCtl_stvHysEngBrkReq,CrCtl_trqLead,CrCtl_trqLimAct,CrCtl_trqMin,CrCtl_trqReq,CrCtl_trqReqOld,CrCtl_vMax
  Bitwise_And{1..12} (12 alike) : simulink/Logic and Bit Operations/Bitwise Operator  logicop=AND  UseBitMask=off  BitMask=bin2dec('11011001')  BitMaskRealWorld=Stored Integer
  Relational Operator1 : RelationalOperator  Operator===  OutDataTypeStr=boolean  RndMeth=Simplest
  Relational Operator2 : RelationalOperator  Operator===  OutDataTypeStr=boolean  RndMeth=Simplest
  Scope : Scope  NumInputPorts=12
  Scope{1..12} (12 alike) : Scope  NumInputPorts=2
  cmp_{1,3..4,6..12} (10 alike) : UnitTest_Lib/RoughlyEqual  slope=0.1
  result_tws : ToWorkspace  VariableName=spec_result_009
  tws_1 : ToWorkspace  VariableName=spec_req_009_001
  tws_10 : ToWorkspace  VariableName=spec_req_009_010
  tws_11 : ToWorkspace  VariableName=spec_req_009_011
  tws_12 : ToWorkspace  VariableName=spec_req_009_012
  tws_2 : ToWorkspace  VariableName=spec_req_009_002
  tws_3 : ToWorkspace  VariableName=spec_req_009_003
  tws_4 : ToWorkspace  VariableName=spec_req_009_004
  tws_5 : ToWorkspace  VariableName=spec_req_009_005
  tws_6 : ToWorkspace  VariableName=spec_req_009_006
  tws_7 : ToWorkspace  VariableName=spec_req_009_007
  tws_8 : ToWorkspace  VariableName=spec_req_009_008
  tws_9 : ToWorkspace  VariableName=spec_req_009_009
  result : Outport
  wires:
  sig_Req_Bus/1 -> BS_Req/1
  sig_Result_Bus/1 -> BS_Result/1
  AndN/1 -> result/1, result_tws/1
  BS_Req/1 -> cmp_1/1, Scope1/1  "<testSig_CrCtl_rTraV2NBeg>"
  BS_Result/1 -> cmp_1/2, Scope1/2  "<CrCtl_rTraV2NBeg>"
  cmp_1/1 -> Bitwise_And1/1
  Bitwise_And1/1 -> AndN/1, Scope/1, tws_1/1
  BS_Req/2 -> Relational Operator1/1, Scope2/1  "<testSig_CrCtl_stOpFunc>"
  BS_Result/2 -> Relational Operator1/2, Scope2/2  "<CrCtl_stOpFunc>"
  Relational Operator1/1 -> Bitwise_And2/1
  Bitwise_And2/1 -> AndN/2, Scope/2, tws_2/1
  BS_Req/3 -> cmp_3/1, Scope3/1  "<testSig_CrCtl_stPtd>"
  BS_Result/3 -> cmp_3/2, Scope3/2  "<CrCtl_stPtd>"
  cmp_3/1 -> Bitwise_And3/1
  Bitwise_And3/1 -> AndN/3, Scope/3, tws_3/1
  BS_Req/4 -> cmp_4/1, Scope4/1  "<testSig_CrCtl_stReq>"
  BS_Result/4 -> cmp_4/2, Scope4/2  "<CrCtl_stReq>"
  cmp_4/1 -> Bitwise_And4/1
  Bitwise_And4/1 -> AndN/4, Scope/4, tws_4/1
  BS_Req/5 -> Relational Operator2/1, Scope5/1  "<testSig_CrCtl_stSuspRamp>"
  BS_Result/5 -> Scope5/2, Relational Operator2/2  "<CrCtl_stSuspRamp>"
  Relational Operator2/1 -> Bitwise_And5/1
  Bitwise_And5/1 -> AndN/5, Scope/5, tws_5/1
  BS_Req/6 -> cmp_6/1, Scope6/1  "<testSig_CrCtl_stvHysEngBrkReq>"
  BS_Result/6 -> cmp_6/2, Scope6/2  "<CrCtl_stvHysEngBrkReq>"
  cmp_6/1 -> Bitwise_And6/1
  Bitwise_And6/1 -> AndN/6, Scope/6, tws_6/1
  BS_Req/7 -> cmp_7/1, Scope7/1  "<testSig_CrCtl_trqLead>"
  BS_Result/7 -> cmp_7/2, Scope7/2  "<CrCtl_trqLead>"
  cmp_7/1 -> Bitwise_And7/1
  Bitwise_And7/1 -> AndN/7, Scope/7, tws_7/1
  BS_Req/8 -> cmp_8/1, Scope8/1  "<testSig_CrCtl_trqLimAct>"
  BS_Result/8 -> cmp_8/2, Scope8/2  "<CrCtl_trqLimAct>"
  cmp_8/1 -> Bitwise_And8/1
  Bitwise_And8/1 -> AndN/8, Scope/8, tws_8/1
  BS_Req/9 -> cmp_9/1, Scope9/1  "<testSig_CrCtl_trqMin>"
  BS_Result/9 -> cmp_9/2, Scope9/2  "<CrCtl_trqMin>"
  cmp_9/1 -> Bitwise_And9/1
  Bitwise_And9/1 -> AndN/9, Scope/9, tws_9/1
  BS_Req/10 -> cmp_10/1, Scope10/1  "<testSig_CrCtl_trqReq>"
  BS_Result/10 -> cmp_10/2, Scope10/2  "<CrCtl_trqReq>"
  cmp_10/1 -> Bitwise_And10/1
  Bitwise_And10/1 -> AndN/10, Scope/10, tws_10/1
  BS_Req/11 -> cmp_11/1, Scope11/1  "<testSig_CrCtl_trqReqOld>"
  BS_Result/11 -> cmp_11/2, Scope11/2  "<CrCtl_trqReqOld>"
  cmp_11/1 -> Bitwise_And11/1
  Bitwise_And11/1 -> AndN/11, Scope/11, tws_11/1
  BS_Req/12 -> cmp_12/1, Scope12/1  "<testSig_CrCtl_vMax>"
  BS_Result/12 -> cmp_12/2, Scope12/2  "<CrCtl_vMax>"
  cmp_12/1 -> Bitwise_And12/1
  Bitwise_And12/1 -> AndN/12, Scope/12, tws_12/1

== system TST_CrCtl_Governor/compareSignals/Requirement_010/specifyOutputs ==
  sig_Req_Bus : Inport
  sig_Result_Bus : Inport  Port=2
  AndN : Logic  Inputs=12
  BS_Req : BusSelector  OutputSignals=testSig_CrCtl_rTraV2NBeg,testSig_CrCtl_stOpFunc,testSig_CrCtl_stPtd,testSig_CrCtl_stReq,testSig_CrCtl_stSuspRamp,testSig_CrCtl_stvHysEngBrkReq,testSig_CrCtl_trqLead,testSig_CrCtl_trqLimAct,testSig_CrCtl_trqMin,testSig_CrCtl_trqReq,testSig_CrCtl_trqReqOld,testSig_CrCtl_vMax
  BS_Result : BusSelector  OutputSignals=CrCtl_rTraV2NBeg,CrCtl_stOpFunc,CrCtl_stPtd,CrCtl_stReq,CrCtl_stSuspRamp,CrCtl_stvHysEngBrkReq,CrCtl_trqLead,CrCtl_trqLimAct,CrCtl_trqMin,CrCtl_trqReq,CrCtl_trqReqOld,CrCtl_vMax
  Bitwise_And{1..12} (12 alike) : simulink/Logic and Bit Operations/Bitwise Operator  logicop=AND  UseBitMask=off  BitMask=bin2dec('11011001')  BitMaskRealWorld=Stored Integer
  Relational Operator1 : RelationalOperator  Operator===  OutDataTypeStr=boolean  RndMeth=Simplest
  Relational Operator2 : RelationalOperator  Operator===  OutDataTypeStr=boolean  RndMeth=Simplest
  Scope : Scope  NumInputPorts=12
  Scope{1..12} (12 alike) : Scope  NumInputPorts=2
  cmp_{1,3..4,6..12} (10 alike) : UnitTest_Lib/RoughlyEqual  slope=0.1
  result_tws : ToWorkspace  VariableName=spec_result_010
  tws_1 : ToWorkspace  VariableName=spec_req_010_001
  tws_10 : ToWorkspace  VariableName=spec_req_010_010
  tws_11 : ToWorkspace  VariableName=spec_req_010_011
  tws_12 : ToWorkspace  VariableName=spec_req_010_012
  tws_2 : ToWorkspace  VariableName=spec_req_010_002
  tws_3 : ToWorkspace  VariableName=spec_req_010_003
  tws_4 : ToWorkspace  VariableName=spec_req_010_004
  tws_5 : ToWorkspace  VariableName=spec_req_010_005
  tws_6 : ToWorkspace  VariableName=spec_req_010_006
  tws_7 : ToWorkspace  VariableName=spec_req_010_007
  tws_8 : ToWorkspace  VariableName=spec_req_010_008
  tws_9 : ToWorkspace  VariableName=spec_req_010_009
  result : Outport
  wires:
  sig_Req_Bus/1 -> BS_Req/1
  sig_Result_Bus/1 -> BS_Result/1
  AndN/1 -> result/1, result_tws/1
  BS_Req/1 -> cmp_1/1, Scope1/1  "<testSig_CrCtl_rTraV2NBeg>"
  BS_Result/1 -> cmp_1/2, Scope1/2  "<CrCtl_rTraV2NBeg>"
  cmp_1/1 -> Bitwise_And1/1
  Bitwise_And1/1 -> AndN/1, Scope/1, tws_1/1
  BS_Req/2 -> Relational Operator1/1, Scope2/1  "<testSig_CrCtl_stOpFunc>"
  BS_Result/2 -> Relational Operator1/2, Scope2/2  "<CrCtl_stOpFunc>"
  Relational Operator1/1 -> Bitwise_And2/1
  Bitwise_And2/1 -> AndN/2, Scope/2, tws_2/1
  BS_Req/3 -> cmp_3/1, Scope3/1  "<testSig_CrCtl_stPtd>"
  BS_Result/3 -> cmp_3/2, Scope3/2  "<CrCtl_stPtd>"
  cmp_3/1 -> Bitwise_And3/1
  Bitwise_And3/1 -> AndN/3, Scope/3, tws_3/1
  BS_Req/4 -> cmp_4/1, Scope4/1  "<testSig_CrCtl_stReq>"
  BS_Result/4 -> cmp_4/2, Scope4/2  "<CrCtl_stReq>"
  cmp_4/1 -> Bitwise_And4/1
  Bitwise_And4/1 -> AndN/4, Scope/4, tws_4/1
  BS_Req/5 -> Relational Operator2/1, Scope5/1  "<testSig_CrCtl_stSuspRamp>"
  BS_Result/5 -> Relational Operator2/2, Scope5/2  "<CrCtl_stSuspRamp>"
  Relational Operator2/1 -> Bitwise_And5/1
  Bitwise_And5/1 -> AndN/5, Scope/5, tws_5/1
  BS_Req/6 -> cmp_6/1, Scope6/1  "<testSig_CrCtl_stvHysEngBrkReq>"
  BS_Result/6 -> cmp_6/2, Scope6/2  "<CrCtl_stvHysEngBrkReq>"
  cmp_6/1 -> Bitwise_And6/1
  Bitwise_And6/1 -> AndN/6, Scope/6, tws_6/1
  BS_Req/7 -> cmp_7/1, Scope7/1  "<testSig_CrCtl_trqLead>"
  BS_Result/7 -> cmp_7/2, Scope7/2  "<CrCtl_trqLead>"
  cmp_7/1 -> Bitwise_And7/1
  Bitwise_And7/1 -> AndN/7, Scope/7, tws_7/1
  BS_Req/8 -> cmp_8/1, Scope8/1  "<testSig_CrCtl_trqLimAct>"
  BS_Result/8 -> cmp_8/2, Scope8/2  "<CrCtl_trqLimAct>"
  cmp_8/1 -> Bitwise_And8/1
  Bitwise_And8/1 -> AndN/8, Scope/8, tws_8/1
  BS_Req/9 -> cmp_9/1, Scope9/1  "<testSig_CrCtl_trqMin>"
  BS_Result/9 -> cmp_9/2, Scope9/2  "<CrCtl_trqMin>"
  cmp_9/1 -> Bitwise_And9/1
  Bitwise_And9/1 -> AndN/9, Scope/9, tws_9/1
  BS_Req/10 -> cmp_10/1, Scope10/1  "<testSig_CrCtl_trqReq>"
  BS_Result/10 -> cmp_10/2, Scope10/2  "<CrCtl_trqReq>"
  cmp_10/1 -> Bitwise_And10/1
  Bitwise_And10/1 -> AndN/10, Scope/10, tws_10/1
  BS_Req/11 -> cmp_11/1, Scope11/1  "<testSig_CrCtl_trqReqOld>"
  BS_Result/11 -> cmp_11/2, Scope11/2  "<CrCtl_trqReqOld>"
  cmp_11/1 -> Bitwise_And11/1
  Bitwise_And11/1 -> AndN/11, Scope/11, tws_11/1
  BS_Req/12 -> cmp_12/1, Scope12/1  "<testSig_CrCtl_vMax>"
  BS_Result/12 -> cmp_12/2, Scope12/2  "<CrCtl_vMax>"
  cmp_12/1 -> Bitwise_And12/1
  Bitwise_And12/1 -> AndN/12, Scope/12, tws_12/1

== system TST_CrCtl_Governor/compareSignals/Requirement_011/specifyOutputs ==
  sig_Req_Bus : Inport
  sig_Result_Bus : Inport  Port=2
  AndN : Logic  Inputs=12
  BS_Req : BusSelector  OutputSignals=testSig_CrCtl_rTraV2NBeg,testSig_CrCtl_stOpFunc,testSig_CrCtl_stPtd,testSig_CrCtl_stReq,testSig_CrCtl_stSuspRamp,testSig_CrCtl_stvHysEngBrkReq,testSig_CrCtl_trqLead,testSig_CrCtl_trqLimAct,testSig_CrCtl_trqMin,testSig_CrCtl_trqReq,testSig_CrCtl_trqReqOld,testSig_CrCtl_vMax
  BS_Result : BusSelector  OutputSignals=CrCtl_rTraV2NBeg,CrCtl_stOpFunc,CrCtl_stPtd,CrCtl_stReq,CrCtl_stSuspRamp,CrCtl_stvHysEngBrkReq,CrCtl_trqLead,CrCtl_trqLimAct,CrCtl_trqMin,CrCtl_trqReq,CrCtl_trqReqOld,CrCtl_vMax
  Bitwise_And{1..12} (12 alike) : simulink/Logic and Bit Operations/Bitwise Operator  logicop=AND  UseBitMask=off  BitMask=bin2dec('11011001')  BitMaskRealWorld=Stored Integer
  Relational Operator1 : RelationalOperator  Operator===  OutDataTypeStr=boolean  RndMeth=Simplest
  Relational Operator2 : RelationalOperator  Operator===  OutDataTypeStr=boolean  RndMeth=Simplest
  Scope : Scope  NumInputPorts=12
  Scope{1..12} (12 alike) : Scope  NumInputPorts=2
  cmp_{1,3..4,6..12} (10 alike) : UnitTest_Lib/RoughlyEqual  slope=0.1
  result_tws : ToWorkspace  VariableName=spec_result_011
  tws_1 : ToWorkspace  VariableName=spec_req_011_001
  tws_10 : ToWorkspace  VariableName=spec_req_011_010
  tws_11 : ToWorkspace  VariableName=spec_req_011_011
  tws_12 : ToWorkspace  VariableName=spec_req_011_012
  tws_2 : ToWorkspace  VariableName=spec_req_011_002
  tws_3 : ToWorkspace  VariableName=spec_req_011_003
  tws_4 : ToWorkspace  VariableName=spec_req_011_004
  tws_5 : ToWorkspace  VariableName=spec_req_011_005
  tws_6 : ToWorkspace  VariableName=spec_req_011_006
  tws_7 : ToWorkspace  VariableName=spec_req_011_007
  tws_8 : ToWorkspace  VariableName=spec_req_011_008
  tws_9 : ToWorkspace  VariableName=spec_req_011_009
  result : Outport
  wires:
  sig_Req_Bus/1 -> BS_Req/1
  sig_Result_Bus/1 -> BS_Result/1
  AndN/1 -> result/1, result_tws/1
  BS_Req/1 -> cmp_1/1, Scope1/1  "<testSig_CrCtl_rTraV2NBeg>"
  BS_Result/1 -> cmp_1/2, Scope1/2  "<CrCtl_rTraV2NBeg>"
  cmp_1/1 -> Bitwise_And1/1
  Bitwise_And1/1 -> AndN/1, Scope/1, tws_1/1
  BS_Req/2 -> Relational Operator1/1, Scope2/1  "<testSig_CrCtl_stOpFunc>"
  BS_Result/2 -> Scope2/2, Relational Operator1/2  "<CrCtl_stOpFunc>"
  Relational Operator1/1 -> Bitwise_And2/1
  Bitwise_And2/1 -> AndN/2, Scope/2, tws_2/1
  BS_Req/3 -> cmp_3/1, Scope3/1  "<testSig_CrCtl_stPtd>"
  BS_Result/3 -> cmp_3/2, Scope3/2  "<CrCtl_stPtd>"
  cmp_3/1 -> Bitwise_And3/1
  Bitwise_And3/1 -> AndN/3, Scope/3, tws_3/1
  BS_Req/4 -> cmp_4/1, Scope4/1  "<testSig_CrCtl_stReq>"
  BS_Result/4 -> cmp_4/2, Scope4/2  "<CrCtl_stReq>"
  cmp_4/1 -> Bitwise_And4/1
  Bitwise_And4/1 -> AndN/4, Scope/4, tws_4/1
  BS_Req/5 -> Relational Operator2/1, Scope5/1  "<testSig_CrCtl_stSuspRamp>"
  BS_Result/5 -> Scope5/2, Relational Operator2/2  "<CrCtl_stSuspRamp>"
  Relational Operator2/1 -> Bitwise_And5/1
  Bitwise_And5/1 -> AndN/5, Scope/5, tws_5/1
  BS_Req/6 -> cmp_6/1, Scope6/1  "<testSig_CrCtl_stvHysEngBrkReq>"
  BS_Result/6 -> cmp_6/2, Scope6/2  "<CrCtl_stvHysEngBrkReq>"
  cmp_6/1 -> Bitwise_And6/1
  Bitwise_And6/1 -> AndN/6, Scope/6, tws_6/1
  BS_Req/7 -> cmp_7/1, Scope7/1  "<testSig_CrCtl_trqLead>"
  BS_Result/7 -> cmp_7/2, Scope7/2  "<CrCtl_trqLead>"
  cmp_7/1 -> Bitwise_And7/1
  Bitwise_And7/1 -> AndN/7, Scope/7, tws_7/1
  BS_Req/8 -> cmp_8/1, Scope8/1  "<testSig_CrCtl_trqLimAct>"
  BS_Result/8 -> cmp_8/2, Scope8/2  "<CrCtl_trqLimAct>"
  cmp_8/1 -> Bitwise_And8/1
  Bitwise_And8/1 -> AndN/8, Scope/8, tws_8/1
  BS_Req/9 -> cmp_9/1, Scope9/1  "<testSig_CrCtl_trqMin>"
  BS_Result/9 -> cmp_9/2, Scope9/2  "<CrCtl_trqMin>"
  cmp_9/1 -> Bitwise_And9/1
  Bitwise_And9/1 -> AndN/9, Scope/9, tws_9/1
  BS_Req/10 -> cmp_10/1, Scope10/1  "<testSig_CrCtl_trqReq>"
  BS_Result/10 -> cmp_10/2, Scope10/2  "<CrCtl_trqReq>"
  cmp_10/1 -> Bitwise_And10/1
  Bitwise_And10/1 -> AndN/10, Scope/10, tws_10/1
  BS_Req/11 -> cmp_11/1, Scope11/1  "<testSig_CrCtl_trqReqOld>"
  BS_Result/11 -> cmp_11/2, Scope11/2  "<CrCtl_trqReqOld>"
  cmp_11/1 -> Bitwise_And11/1
  Bitwise_And11/1 -> AndN/11, Scope/11, tws_11/1
  BS_Req/12 -> cmp_12/1, Scope12/1  "<testSig_CrCtl_vMax>"
  BS_Result/12 -> cmp_12/2, Scope12/2  "<CrCtl_vMax>"
  cmp_12/1 -> Bitwise_And12/1
  Bitwise_And12/1 -> AndN/12, Scope/12, tws_12/1
